simulink model "Question_5"  (R2014a)
settings: Solver=ode45  StartTime=0.0  StopTime=10.0  RelTol=1e-3
libraries: hdlsllib x4
settings Model: Creator=Shiyu  LastModifiedBy=Shiyu

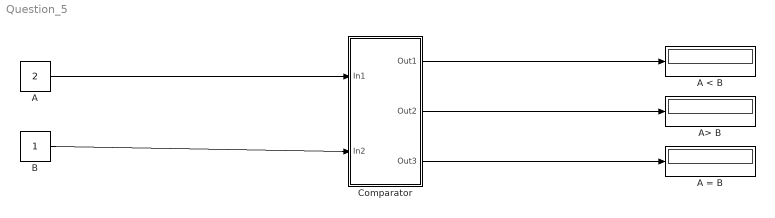
== system Question_5 ==
  A : Constant  Value=2  OutMin=[0]  OutMax=[3]  OutDataTypeStr=uint8
  A < B : Display
  A = B : Display
  A> B : Display
  B : Constant  OutMin=[0]  OutMax=[3]  OutDataTypeStr=uint8
  "Comparator " : Subsystem
  wires:
  A/1 -> "Comparator "/1(In1)
  B/1 -> "Comparator "/2(In2)
  "Comparator "/1(Out1) -> A < B/1
  "Comparator "/2(Out2) -> A> B/1
  "Comparator "/3(Out3) -> A = B/1

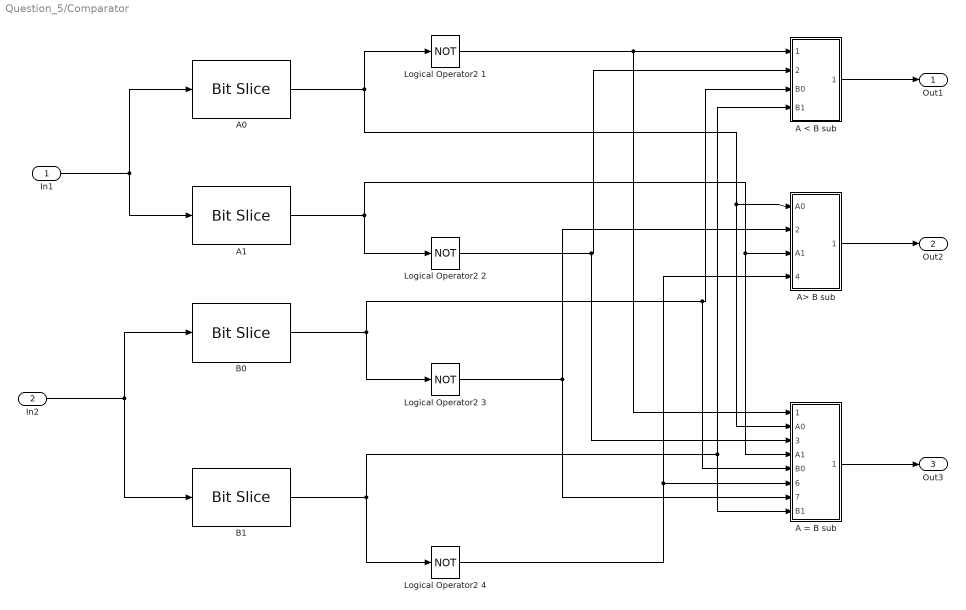
== system Question_5/Comparator  ==
  In1 : Inport  OutDataTypeStr=uint8  SampleTime=1
  In2 : Inport  Port=2  OutDataTypeStr=uint8  SampleTime=1
  "A < B sub " : Subsystem
  "A = B sub " : Subsystem
  A0 : hdlsllib/HDL Operations/Bit Slice  lidx=1  ridx=1
  A1 : hdlsllib/HDL Operations/Bit Slice  lidx=0  ridx=0
  A> B sub : Subsystem
  B0 : hdlsllib/HDL Operations/Bit Slice  lidx=1  ridx=1
  B1 : hdlsllib/HDL Operations/Bit Slice  lidx=0  ridx=0
  Logical Operator2 {1..4} (4 alike) : Logic  Operator=NOT  Inputs=3  AllPortsSameDT=off  OutDataTypeStr=boolean
  Out1 : Outport
  Out2 : Outport  Port=2
  Out3 : Outport  Port=3
  wires:
  B1/1 -> "A < B sub "/4(B1), "A = B sub "/8(B1), Logical Operator2 4/1
  "A < B sub "/1(Out2) -> Out1/1
  Logical Operator2 1/1 -> "A = B sub "/1(~A0), "A < B sub "/1(~A0)
  Logical Operator2 2/1 -> "A = B sub "/3(~A1), "A < B sub "/2(~A1)
  B0/1 -> "A = B sub "/5(B0), "A < B sub "/3(B0), Logical Operator2 3/1
  Logical Operator2 3/1 -> "A = B sub "/7(~B0), A> B sub/2(~B0)
  A0/1 -> "A = B sub "/2(A0), A> B sub/1(A0), Logical Operator2 1/1
  A1/1 -> Logical Operator2 2/1, "A = B sub "/4(A1), A> B sub/3(A1)
  In1/1 -> A1/1, A0/1
  In2/1 -> B0/1, B1/1
  Logical Operator2 4/1 -> A> B sub/4(~B1), "A = B sub "/6(~B1)
  A> B sub/1(Out1) -> Out2/1
  "A = B sub "/1(Out4) -> Out3/1

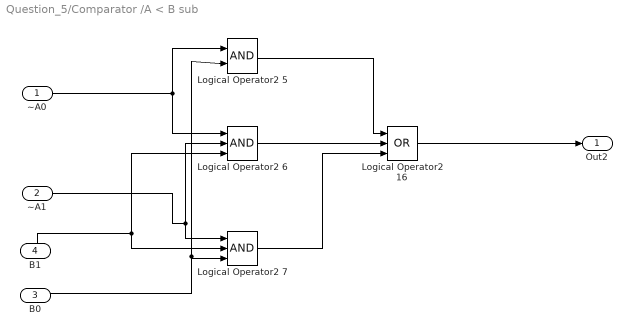
== system Question_5/Comparator /A < B sub  ==
  ~A0 : Inport
  ~A1 : Inport  Port=2
  B0 : Inport  Port=3
  B1 : Inport  Port=4
  Logical Operator2 16 : Logic  Operator=OR  Inputs=3  AllPortsSameDT=off  OutDataTypeStr=boolean
  Logical Operator2 5 : Logic  AllPortsSameDT=off  OutDataTypeStr=boolean
  Logical Operator2 6 : Logic  Inputs=3  AllPortsSameDT=off  OutDataTypeStr=boolean
  Logical Operator2 7 : Logic  Inputs=3  AllPortsSameDT=off  OutDataTypeStr=boolean
  Out2 : Outport
  wires:
  ~A1/1 -> Logical Operator2 6/2, Logical Operator2 7/1
  ~A0/1 -> Logical Operator2 6/1, Logical Operator2 5/1
  B1/1 -> Logical Operator2 7/2, Logical Operator2 6/3
  B0/1 -> Logical Operator2 5/2, Logical Operator2 7/3
  Logical Operator2 7/1 -> Logical Operator2 16/3
  Logical Operator2 16/1 -> Out2/1
  Logical Operator2 6/1 -> Logical Operator2 16/2
  Logical Operator2 5/1 -> Logical Operator2 16/1

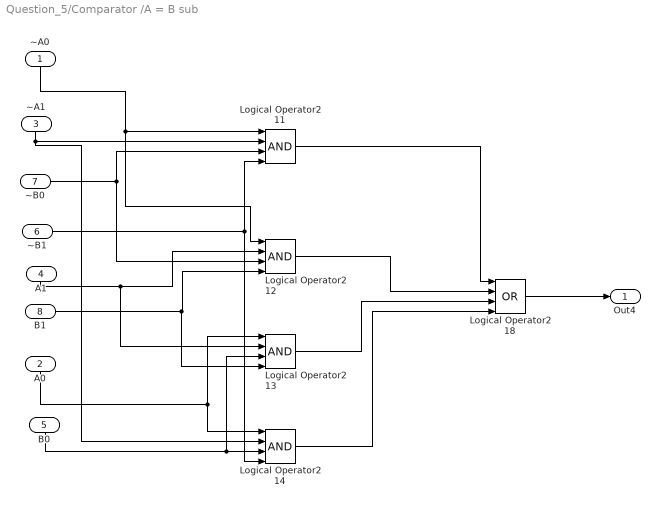
== system Question_5/Comparator /A = B sub  ==
  ~A0 : Inport
  A0 : Inport  Port=2
  ~A1 : Inport  Port=3
  A1 : Inport  Port=4
  B0 : Inport  Port=5
  ~B1 : Inport  Port=6
  ~B0 : Inport  Port=7
  B1 : Inport  Port=8
  Logical Operator2 {11..14} (4 alike) : Logic  Inputs=4  AllPortsSameDT=off  OutDataTypeStr=boolean
  Logical Operator2 18 : Logic  Operator=OR  Inputs=4  AllPortsSameDT=off  OutDataTypeStr=boolean
  Out4 : Outport
  wires:
  Logical Operator2 18/1 -> Out4/1
  Logical Operator2 12/1 -> Logical Operator2 18/2
  Logical Operator2 13/1 -> Logical Operator2 18/3
  Logical Operator2 14/1 -> Logical Operator2 18/4
  Logical Operator2 11/1 -> Logical Operator2 18/1
  ~A0/1 -> Logical Operator2 12/1, Logical Operator2 11/1
  B0/1 -> Logical Operator2 14/3, Logical Operator2 13/3
  ~B1/1 -> Logical Operator2 11/4, Logical Operator2 14/4
  B1/1 -> Logical Operator2 13/4, Logical Operator2 12/4
  ~A1/1 -> Logical Operator2 14/2, Logical Operator2 11/2
  ~B0/1 -> Logical Operator2 11/3, Logical Operator2 12/3
  A1/1 -> Logical Operator2 13/2, Logical Operator2 12/2
  A0/1 -> Logical Operator2 14/1, Logical Operator2 13/1

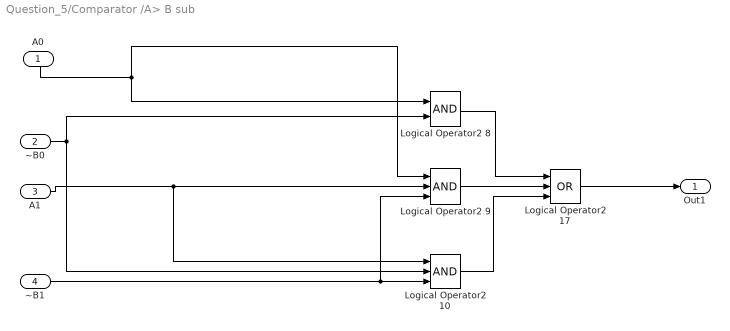
== system Question_5/Comparator /A> B sub ==
  A0 : Inport
  ~B0 : Inport  Port=2
  A1 : Inport  Port=3
  ~B1 : Inport  Port=4
  Logical Operator2 10 : Logic  Inputs=3  AllPortsSameDT=off  OutDataTypeStr=boolean
  Logical Operator2 17 : Logic  Operator=OR  Inputs=3  AllPortsSameDT=off  OutDataTypeStr=boolean
  Logical Operator2 8 : Logic  AllPortsSameDT=off  OutDataTypeStr=boolean
  Logical Operator2 9 : Logic  Inputs=3  AllPortsSameDT=off  OutDataTypeStr=boolean
  Out1 : Outport
  wires:
  Logical Operator2 17/1 -> Out1/1
  Logical Operator2 8/1 -> Logical Operator2 17/1
  ~B1/1 -> Logical Operator2 9/3, Logical Operator2 10/3
  Logical Operator2 9/1 -> Logical Operator2 17/2
  A1/1 -> Logical Operator2 10/1, Logical Operator2 9/2
  ~B0/1 -> Logical Operator2 8/2, Logical Operator2 10/2
  A0/1 -> Logical Operator2 9/1, Logical Operator2 8/1
  Logical Operator2 10/1 -> Logical Operator2 17/3
